simulink model "BlockDiagram_DCmotor_noControl"  (R2019a)
settings: Solver=VariableStepAuto  StartTime=0.0  StopTime=500.0  RelTol=1e-3
values from neighbouring files (symbols this model uses):
  Jeq = 1    [DCmotor_InputData.m]    (also in DCmotor_InputData_lecture20.m = 0.0022; DCmotor_InputData_lecture20_control1.m = 0.0022; DCmotor_InputData_lecture20_control_study.m = 0.0022; DCmotor_InputData_lecture20_loadLin.m = 0.0022)
  kE = 0.5    [DCmotor_InputData.m]    (also in DCmotor_InputData_lecture20.m = 0.129; DCmotor_InputData_lecture20_control1.m = 0.129; DCmotor_InputData_lecture20_control_study.m = 0.129; DCmotor_InputData_lecture20_loadLin.m = 0.129)
  kT = 0.5    [DCmotor_InputData.m]    (also in DCmotor_InputData_lecture20.m = 0.129; DCmotor_InputData_lecture20_control1.m = 0.129; DCmotor_InputData_lecture20_control_study.m = 0.129; DCmotor_InputData_lecture20_loadLin.m = 0.129)
  La = 0.2    [DCmotor_InputData.m]    (also in DCmotor_InputData_lecture20.m = 0.0072; DCmotor_InputData_lecture20_control1.m = 0.0072; DCmotor_InputData_lecture20_control_study.m = 0.0072; DCmotor_InputData_lecture20_loadLin.m = 0.0072)
  Ra = 0.02    [DCmotor_InputData.m]    (also in DCmotor_InputData_lecture20.m = 0.5; DCmotor_InputData_lecture20_control1.m = 0.5; DCmotor_InputData_lecture20_control_study.m = 0.5; DCmotor_InputData_lecture20_loadLin.m = 0.5)
settings Model: Creator=Luca Papini  LastModifiedBy=Luca Papini
settings DataIOCC: SaveFormat=StructureWithTime  SaveState=on

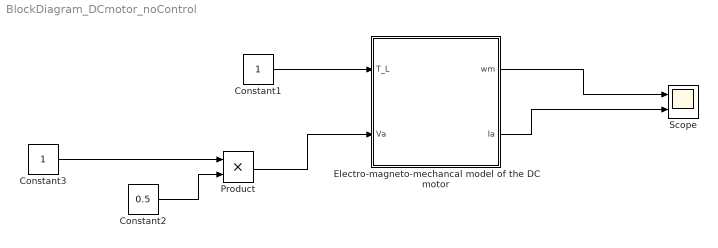
== system BlockDiagram_DCmotor_noControl ==
  Constant1 : Constant
  Constant2 : Constant  Value=0.5
  Constant3 : Constant
  Electro-magneto-mechancal model of the DC motor : Subsystem
  Product : Product
  Scope : Scope  NumInputPorts=2
  wires:
  Electro-magneto-mechancal model of the DC motor/1(wm) -> Scope/1
  Electro-magneto-mechancal model of the DC motor/2(Ia) -> Scope/2
  Constant1/1 -> Electro-magneto-mechancal model of the DC motor/1(T_L)
  Product/1 -> Electro-magneto-mechancal model of the DC motor/2(Va)
  Constant2/1 -> Product/2
  Constant3/1 -> Product/1

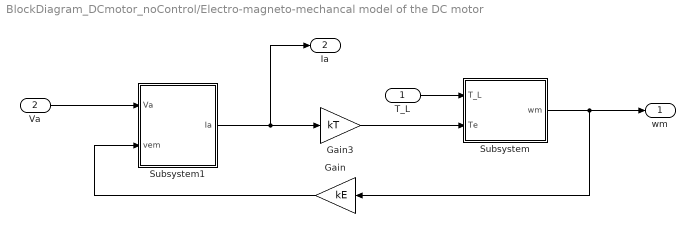
== system BlockDiagram_DCmotor_noControl/Electro-magneto-mechancal model of the DC motor ==
  T_L : Inport
  Va : Inport  Port=2
  Gain : Gain  Gain=kE
  Gain3 : Gain  Gain=kT
  Subsystem : Subsystem
  Subsystem1 : Subsystem
  wm : Outport
  Ia : Outport  Port=2
  wires:
  Va/1 -> Subsystem1/1(Va)
  Gain3/1 -> Subsystem/2(Te)
  Subsystem/1(wm) -> Gain/1, wm/1
  Gain/1 -> Subsystem1/2(vem)
  Subsystem1/1(Ia) -> Ia/1, Gain3/1
  T_L/1 -> Subsystem/1(T_L)

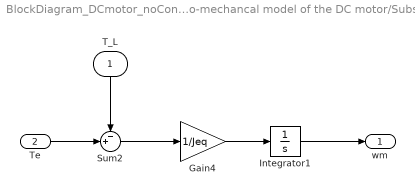
== system BlockDiagram_DCmotor_noControl/Electro-magneto-mechancal model of the DC motor/Subsystem ==
  T_L : Inport
  Te : Inport  Port=2
  Gain4 : Gain  Gain=1/Jeq
  Integrator1 : Integrator
  Sum2 : Sum  Inputs=-+|
  wm : Outport
  wires:
  Sum2/1 -> Gain4/1
  Integrator1/1 -> wm/1
  T_L/1 -> Sum2/1
  Gain4/1 -> Integrator1/1
  Te/1 -> Sum2/2

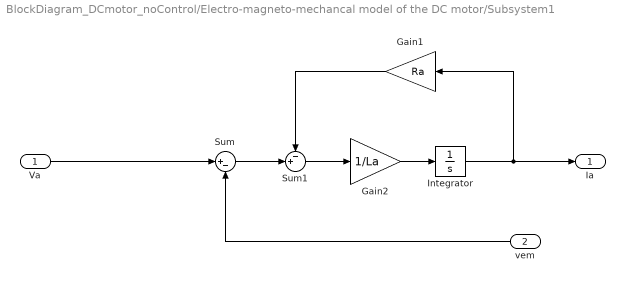
== system BlockDiagram_DCmotor_noControl/Electro-magneto-mechancal model of the DC motor/Subsystem1 ==
  Va : Inport
  vem : Inport  Port=2
  Gain1 : Gain  Gain=Ra
  Gain2 : Gain  Gain=1/La
  Integrator : Integrator
  Sum : Sum  Inputs=|+-
  Sum1 : Sum  Inputs=-+|
  Ia : Outport
  wires:
  Integrator/1 -> Ia/1, Gain1/1
  Gain2/1 -> Integrator/1
  Va/1 -> Sum/1
  Sum1/1 -> Gain2/1
  Gain1/1 -> Sum1/1
  vem/1 -> Sum/2
  Sum/1 -> Sum1/2
